simulink library "csc_valvesim_collection_lib"  (R2014b)
settings: Solver=ode45  StartTime=0.0  StopTime=10.0  RelTol=1e-3
libraries: csc_valvesim_sim_lib x26
settings Model: Creator=escrane  LastModifiedBy=mstewart

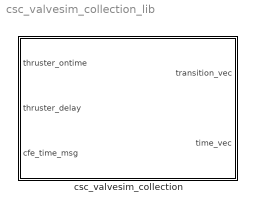
== system csc_valvesim_collection_lib ==
  csc_valvesim_collection : Subsystem
      mask Display: color('blue');text(0.05, 0.02, 'MoonEx', 'HorizontalAlignment', 'Left', 'VerticalAlignment', 'Bottom');color('red');text(0.95, 0.02, 'Autogenerated', 'HorizontalAlignment', 'Right', 'VerticalAlignment', 'Bottom');

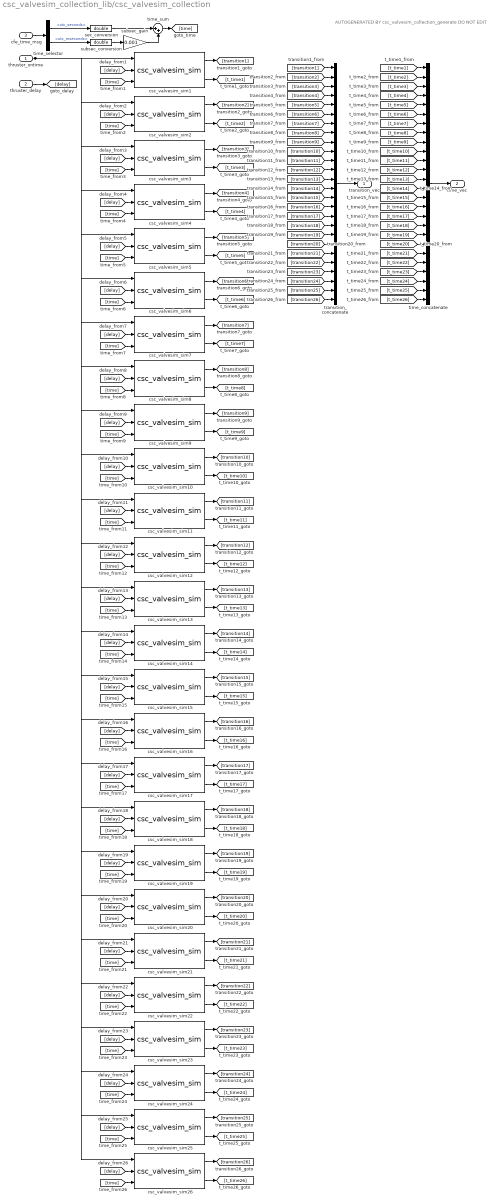
== system csc_valvesim_collection_lib/csc_valvesim_collection ==
  note: AUTOGENERATED BY csc_valvesim_collection_generate
      | DO NOT EDIT
  thruster_ontime : Inport
  thruster_delay : Inport  Port=2
  cfe_time_msg : Inport  Port=3
  csc_valvesim_sim1 : csc_valvesim_sim_lib/csc_valvesim_sim  thruster_idx=1  num_thrusters=26
  csc_valvesim_sim10 : csc_valvesim_sim_lib/csc_valvesim_sim  thruster_idx=10  num_thrusters=26
  csc_valvesim_sim11 : csc_valvesim_sim_lib/csc_valvesim_sim  thruster_idx=11  num_thrusters=26
  csc_valvesim_sim12 : csc_valvesim_sim_lib/csc_valvesim_sim  thruster_idx=12  num_thrusters=26
  csc_valvesim_sim13 : csc_valvesim_sim_lib/csc_valvesim_sim  thruster_idx=13  num_thrusters=26
  csc_valvesim_sim14 : csc_valvesim_sim_lib/csc_valvesim_sim  thruster_idx=14  num_thrusters=26
  csc_valvesim_sim15 : csc_valvesim_sim_lib/csc_valvesim_sim  thruster_idx=15  num_thrusters=26
  csc_valvesim_sim16 : csc_valvesim_sim_lib/csc_valvesim_sim  thruster_idx=16  num_thrusters=26
  csc_valvesim_sim17 : csc_valvesim_sim_lib/csc_valvesim_sim  thruster_idx=17  num_thrusters=26
  csc_valvesim_sim18 : csc_valvesim_sim_lib/csc_valvesim_sim  thruster_idx=18  num_thrusters=26
  csc_valvesim_sim19 : csc_valvesim_sim_lib/csc_valvesim_sim  thruster_idx=19  num_thrusters=26
  csc_valvesim_sim2 : csc_valvesim_sim_lib/csc_valvesim_sim  thruster_idx=2  num_thrusters=26
  csc_valvesim_sim20 : csc_valvesim_sim_lib/csc_valvesim_sim  thruster_idx=20  num_thrusters=26
  csc_valvesim_sim21 : csc_valvesim_sim_lib/csc_valvesim_sim  thruster_idx=21  num_thrusters=26
  csc_valvesim_sim22 : csc_valvesim_sim_lib/csc_valvesim_sim  thruster_idx=22  num_thrusters=26
  csc_valvesim_sim23 : csc_valvesim_sim_lib/csc_valvesim_sim  thruster_idx=23  num_thrusters=26
  csc_valvesim_sim24 : csc_valvesim_sim_lib/csc_valvesim_sim  thruster_idx=24  num_thrusters=26
  csc_valvesim_sim25 : csc_valvesim_sim_lib/csc_valvesim_sim  thruster_idx=25  num_thrusters=26
  csc_valvesim_sim26 : csc_valvesim_sim_lib/csc_valvesim_sim  thruster_idx=26  num_thrusters=26
  csc_valvesim_sim3 : csc_valvesim_sim_lib/csc_valvesim_sim  thruster_idx=3  num_thrusters=26
  csc_valvesim_sim4 : csc_valvesim_sim_lib/csc_valvesim_sim  thruster_idx=4  num_thrusters=26
  csc_valvesim_sim5 : csc_valvesim_sim_lib/csc_valvesim_sim  thruster_idx=5  num_thrusters=26
  csc_valvesim_sim6 : csc_valvesim_sim_lib/csc_valvesim_sim  thruster_idx=6  num_thrusters=26
  csc_valvesim_sim7 : csc_valvesim_sim_lib/csc_valvesim_sim  thruster_idx=7  num_thrusters=26
  csc_valvesim_sim8 : csc_valvesim_sim_lib/csc_valvesim_sim  thruster_idx=8  num_thrusters=26
  csc_valvesim_sim9 : csc_valvesim_sim_lib/csc_valvesim_sim  thruster_idx=9  num_thrusters=26
  sec_conversion : DataTypeConversion  OutDataTypeStr=double  SaturateOnIntegerOverflow=on  RndMeth=Zero
  subsec_conversion : DataTypeConversion  OutDataTypeStr=double  SaturateOnIntegerOverflow=on  RndMeth=Zero
  subsec_gain : Gain  Gain=0.001  SaturateOnIntegerOverflow=on  OutDataTypeStr=Inherit: Same as input  ParamDataTypeStr=Inherit: Same as input
  time_concatenate : Concatenate  NumInputs=26
  time_selector : BusSelector  OutputSignals=utc_seconds,utc_mseconds
  time_sum : Sum  Inputs=|++  SaturateOnIntegerOverflow=on  InputSameDT=on  OutDataTypeStr=Inherit: Same as first input
  transition_concatenate : Concatenate  NumInputs=26
  transition_vec : Outport
  time_vec : Outport  Port=2
  wires:
  cfe_time_msg/1 -> time_selector/1
  time_selector/1 -> sec_conversion/1  "<utc_seconds>"
  time_selector/2 -> subsec_conversion/1  "<utc_mseconds>"
  subsec_conversion/1 -> subsec_gain/1
  subsec_gain/1 -> time_sum/2
  sec_conversion/1 -> time_sum/1
  time_sum/1 -> [time]
  thruster_delay/1 -> [delay]
  transition_concatenate/1 -> transition_vec/1
  time_concatenate/1 -> time_vec/1
  [transition1] -> transition_concatenate/1
  [t_time1] -> time_concatenate/1
  [delay] -> csc_valvesim_sim1/2
  [time] -> csc_valvesim_sim1/3
  csc_valvesim_sim1/1 -> [transition1]
  csc_valvesim_sim1/2 -> [t_time1]
  [transition2] -> transition_concatenate/2
  [t_time2] -> time_concatenate/2
  [delay] -> csc_valvesim_sim2/2
  [time] -> csc_valvesim_sim2/3
  csc_valvesim_sim2/1 -> [transition2]
  csc_valvesim_sim2/2 -> [t_time2]
  [transition3] -> transition_concatenate/3
  [t_time3] -> time_concatenate/3
  [delay] -> csc_valvesim_sim3/2
  [time] -> csc_valvesim_sim3/3
  csc_valvesim_sim3/1 -> [transition3]
  csc_valvesim_sim3/2 -> [t_time3]
  [transition4] -> transition_concatenate/4
  [t_time4] -> time_concatenate/4
  [delay] -> csc_valvesim_sim4/2
  [time] -> csc_valvesim_sim4/3
  csc_valvesim_sim4/1 -> [transition4]
  csc_valvesim_sim4/2 -> [t_time4]
  [transition5] -> transition_concatenate/5
  [t_time5] -> time_concatenate/5
  [delay] -> csc_valvesim_sim5/2
  [time] -> csc_valvesim_sim5/3
  csc_valvesim_sim5/1 -> [transition5]
  csc_valvesim_sim5/2 -> [t_time5]
  [transition6] -> transition_concatenate/6
  [t_time6] -> time_concatenate/6
  [delay] -> csc_valvesim_sim6/2
  [time] -> csc_valvesim_sim6/3
  csc_valvesim_sim6/1 -> [transition6]
  csc_valvesim_sim6/2 -> [t_time6]
  [transition7] -> transition_concatenate/7
  [t_time7] -> time_concatenate/7
  [delay] -> csc_valvesim_sim7/2
  [time] -> csc_valvesim_sim7/3
  csc_valvesim_sim7/1 -> [transition7]
  csc_valvesim_sim7/2 -> [t_time7]
  [transition8] -> transition_concatenate/8
  [t_time8] -> time_concatenate/8
  [delay] -> csc_valvesim_sim8/2
  [time] -> csc_valvesim_sim8/3
  csc_valvesim_sim8/1 -> [transition8]
  csc_valvesim_sim8/2 -> [t_time8]
  [transition9] -> transition_concatenate/9
  [t_time9] -> time_concatenate/9
  [delay] -> csc_valvesim_sim9/2
  [time] -> csc_valvesim_sim9/3
  csc_valvesim_sim9/1 -> [transition9]
  csc_valvesim_sim9/2 -> [t_time9]
  [transition10] -> transition_concatenate/10
  [t_time10] -> time_concatenate/10
  [delay] -> csc_valvesim_sim10/2
  [time] -> csc_valvesim_sim10/3
  csc_valvesim_sim10/1 -> [transition10]
  csc_valvesim_sim10/2 -> [t_time10]
  [transition11] -> transition_concatenate/11
  [t_time11] -> time_concatenate/11
  [delay] -> csc_valvesim_sim11/2
  [time] -> csc_valvesim_sim11/3
  csc_valvesim_sim11/1 -> [transition11]
  csc_valvesim_sim11/2 -> [t_time11]
  [transition12] -> transition_concatenate/12
  [t_time12] -> time_concatenate/12
  [delay] -> csc_valvesim_sim12/2
  [time] -> csc_valvesim_sim12/3
  csc_valvesim_sim12/1 -> [transition12]
  csc_valvesim_sim12/2 -> [t_time12]
  [transition13] -> transition_concatenate/13
  [t_time13] -> time_concatenate/13
  [delay] -> csc_valvesim_sim13/2
  [time] -> csc_valvesim_sim13/3
  csc_valvesim_sim13/1 -> [transition13]
  csc_valvesim_sim13/2 -> [t_time13]
  [transition14] -> transition_concatenate/14
  [t_time14] -> time_concatenate/14
  [delay] -> csc_valvesim_sim14/2
  [time] -> csc_valvesim_sim14/3
  csc_valvesim_sim14/1 -> [transition14]
  csc_valvesim_sim14/2 -> [t_time14]
  [transition15] -> transition_concatenate/15
  [t_time15] -> time_concatenate/15
  [delay] -> csc_valvesim_sim15/2
  [time] -> csc_valvesim_sim15/3
  csc_valvesim_sim15/1 -> [transition15]
  csc_valvesim_sim15/2 -> [t_time15]
  [transition16] -> transition_concatenate/16
  [t_time16] -> time_concatenate/16
  [delay] -> csc_valvesim_sim16/2
  [time] -> csc_valvesim_sim16/3
  csc_valvesim_sim16/1 -> [transition16]
  csc_valvesim_sim16/2 -> [t_time16]
  [transition17] -> transition_concatenate/17
  [t_time17] -> time_concatenate/17
  [delay] -> csc_valvesim_sim17/2
  [time] -> csc_valvesim_sim17/3
  csc_valvesim_sim17/1 -> [transition17]
  csc_valvesim_sim17/2 -> [t_time17]
  [transition18] -> transition_concatenate/18
  [t_time18] -> time_concatenate/18
  [delay] -> csc_valvesim_sim18/2
  [time] -> csc_valvesim_sim18/3
  csc_valvesim_sim18/1 -> [transition18]
  csc_valvesim_sim18/2 -> [t_time18]
  [transition19] -> transition_concatenate/19
  [t_time19] -> time_concatenate/19
  [delay] -> csc_valvesim_sim19/2
  [time] -> csc_valvesim_sim19/3
  csc_valvesim_sim19/1 -> [transition19]
  csc_valvesim_sim19/2 -> [t_time19]
  [transition20] -> transition_concatenate/20
  [t_time20] -> time_concatenate/20
  [delay] -> csc_valvesim_sim20/2
  [time] -> csc_valvesim_sim20/3
  csc_valvesim_sim20/1 -> [transition20]
  csc_valvesim_sim20/2 -> [t_time20]
  [transition21] -> transition_concatenate/21
  [t_time21] -> time_concatenate/21
  [delay] -> csc_valvesim_sim21/2
  [time] -> csc_valvesim_sim21/3
  csc_valvesim_sim21/1 -> [transition21]
  csc_valvesim_sim21/2 -> [t_time21]
  [transition22] -> transition_concatenate/22
  [t_time22] -> time_concatenate/22
  [delay] -> csc_valvesim_sim22/2
  [time] -> csc_valvesim_sim22/3
  csc_valvesim_sim22/1 -> [transition22]
  csc_valvesim_sim22/2 -> [t_time22]
  [transition23] -> transition_concatenate/23
  [t_time23] -> time_concatenate/23
  [delay] -> csc_valvesim_sim23/2
  [time] -> csc_valvesim_sim23/3
  csc_valvesim_sim23/1 -> [transition23]
  csc_valvesim_sim23/2 -> [t_time23]
  [transition24] -> transition_concatenate/24
  [t_time24] -> time_concatenate/24
  [delay] -> csc_valvesim_sim24/2
  [time] -> csc_valvesim_sim24/3
  csc_valvesim_sim24/1 -> [transition24]
  csc_valvesim_sim24/2 -> [t_time24]
  [transition25] -> transition_concatenate/25
  [t_time25] -> time_concatenate/25
  [delay] -> csc_valvesim_sim25/2
  [time] -> csc_valvesim_sim25/3
  csc_valvesim_sim25/1 -> [transition25]
  csc_valvesim_sim25/2 -> [t_time25]
  [transition26] -> transition_concatenate/26
  [t_time26] -> time_concatenate/26
  [delay] -> csc_valvesim_sim26/2
  [time] -> csc_valvesim_sim26/3
  csc_valvesim_sim26/1 -> [transition26]
  csc_valvesim_sim26/2 -> [t_time26]
  thruster_ontime/1 -> csc_valvesim_sim26/1, csc_valvesim_sim25/1, csc_valvesim_sim24/1, csc_valvesim_sim23/1, csc_valvesim_sim22/1, csc_valvesim_sim21/1, csc_valvesim_sim20/1, csc_valvesim_sim19/1, csc_valvesim_sim18/1, csc_valvesim_sim17/1, csc_valvesim_sim16/1, csc_valvesim_sim15/1, csc_valvesim_sim14/1, csc_valvesim_sim13/1, csc_valvesim_sim12/1, csc_valvesim_sim11/1, csc_valvesim_sim10/1, csc_valvesim_sim9/1, csc_valvesim_sim8/1, csc_valvesim_sim7/1, csc_valvesim_sim6/1, csc_valvesim_sim5/1, csc_valvesim_sim4/1, csc_valvesim_sim3/1, csc_valvesim_sim2/1, csc_valvesim_sim1/1
